simulink model "saturation_mdl"  (R2013b)
settings: Solver=ode45  StartTime=0.0  StopTime=10.0  MaxStep=1e-3  RelTol=1e-3
libraries: cstblocks x4
settings Model: Creator=daniw  LastModifiedBy=daniw

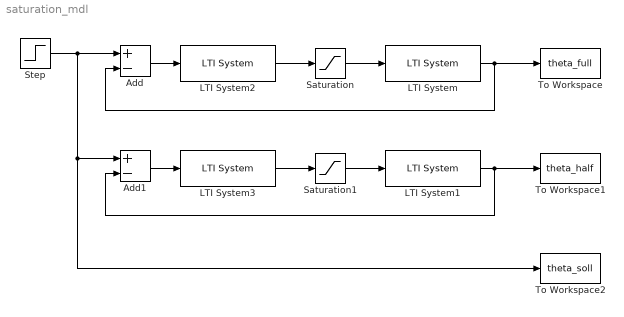
== system saturation_mdl ==
  Add : Sum  Inputs=+-
  Add1 : Sum  Inputs=+-
  LTI System : cstblocks/LTI System  sys=G1_full  IC=[]
  LTI System1 : cstblocks/LTI System  sys=G1_half  IC=[]
  LTI System2 : cstblocks/LTI System  sys=C  IC=[]
  LTI System3 : cstblocks/LTI System  sys=C  IC=[]
  Saturation : Saturate  UpperLimit=10  LowerLimit=0
  Saturation1 : Saturate  UpperLimit=10  LowerLimit=0
  Step : Step  SampleTime=0
  To Workspace : ToWorkspace  VariableName=theta_full  SampleTime=-1  SaveFormat=Structure With Time
  To Workspace1 : ToWorkspace  VariableName=theta_half  SampleTime=-1  SaveFormat=Structure With Time
  To Workspace2 : ToWorkspace  VariableName=theta_soll  SampleTime=-1  SaveFormat=Structure With Time
  wires:
  Step/1 -> To Workspace2/1, Add1/1, Add/1
  Add/1 -> LTI System2/1
  LTI System2/1 -> Saturation/1
  LTI System/1 -> To Workspace/1, Add/2
  Add1/1 -> LTI System3/1
  LTI System3/1 -> Saturation1/1
  LTI System1/1 -> To Workspace1/1, Add1/2
  Saturation/1 -> LTI System/1
  Saturation1/1 -> LTI System1/1
